simulink model "sampleModel1605_4_sub_sub"  (R2023a)
settings: Solver=VariableStepAuto  StartTime=0.0  StopTime=10.0  RelTol=1e-3
libraries: hdlsllib x2
settings Model: Creator=user1  LastModifiedBy=user1

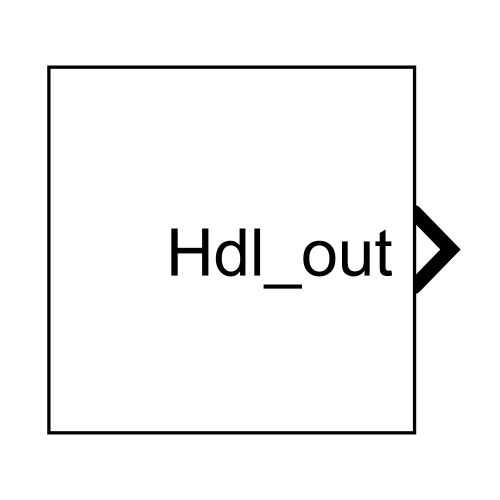
[thumbnail: Simulink's stored preview of the top-level diagram]
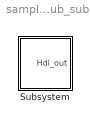
== system sampleModel1605_4_sub_sub ==
  Subsystem : Subsystem

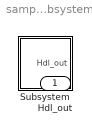
== system sampleModel1605_4_sub_sub/Subsystem ==
  Subsystem : Subsystem
  Hdl_out : Outport  OutDataTypeStr=uint8

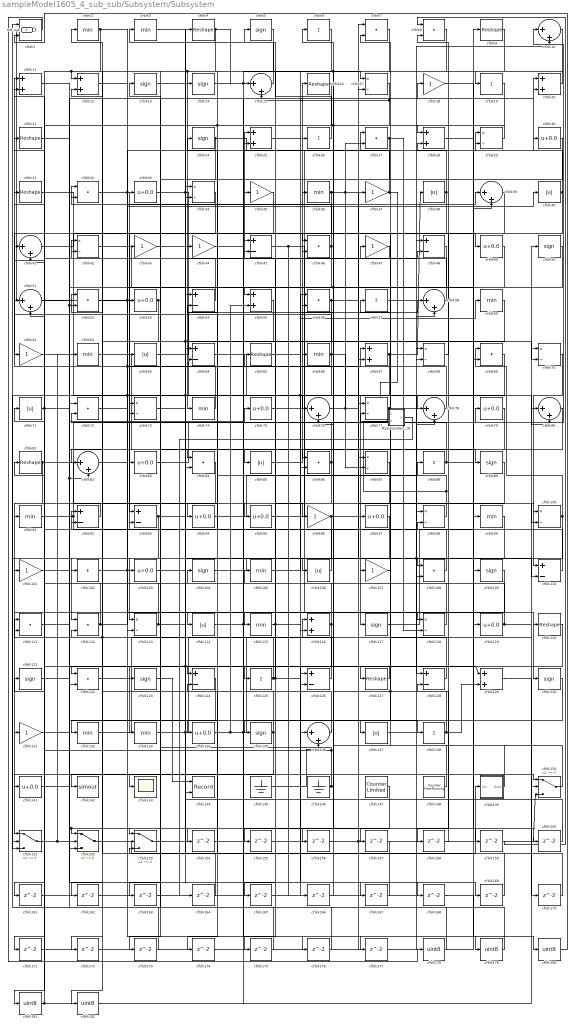
== system sampleModel1605_4_sub_sub/Subsystem/Subsystem ==
  Mysubsystem_16 : Subsystem  TreatAsAtomicUnit=on  RTWFcnName=Mysubsystem_16
      settings: RTWFcnNameOpts=User specified  RTWFileNameOpts=Use function name
  cfblk1 : Logic  AllPortsSameDT=off  OutDataTypeStr=boolean
  cfblk{10,15,39,41,51,58,76,78,80,82,136} (11 alike) : Sum  Inputs=|++  OutDataTypeStr=uint8
  cfblk{17,29,34,42,68,70,73,77,87,98,100,113,118} (13 alike) : Product  Inputs=*/  OutDataTypeStr=uint8  RndMeth=Zero  SaturateOnIntegerOverflow=on
  cfblk{18,35,37,43..44,47,61,96,101,107,131} (11 alike) : Gain  OutDataTypeStr=uint8
  cfblk{6,19,26,57,88,102,125,138} (8 alike) : Sum  Inputs=+  OutDataTypeStr=uint8
  cfblk{30,33,49,53,75,79,83,94..95,97,103,119,134,141} (14 alike) : Bias  Bias=0.0  SaturateOnIntegerOverflow=off
  cfblk{5,13..14,24,50,89,104,109,117,121,123,130,135} (13 alike) : Signum
  cfblk{2..3,36,59,62,66,74,91,99,105,115,132..133} (13 alike) : MinMax  OutDataTypeStr=uint8
  cfblk{38,40,63,71,85,106,114,137} (8 alike) : Abs  OutDataTypeStr=uint8  SaturateOnIntegerOverflow=off
  cfblk{7..8,27,32,46,52,56,69,72,84,86,108,111..112,122} (15 alike) : DotProduct  OutDataTypeStr=uint8
  cfblk{11..12,20,25,28,55,67,116,129} (9 alike) : Sum  OutDataTypeStr=uint8
  cfblk{45,48,54,64,92..93,110,124,126,128} (10 alike) : Sum  Inputs=+-  OutDataTypeStr=uint8
  cfblk{4,9,16,21,31,65,81,120,127} (9 alike) : Reshape
  cfblk142 : ToWorkspace  VariableName=simout  SaveFormat=Timeseries  SampleTime=-1
  cfblk143 : Scope
  cfblk144 : Record  FileSettingsInternal="{\"entries\":[{\"content\":{\"excelSettings\":{\"content\":{},\"type\":\"Streamout.ExcelSettings\"}},\"type\":\"Streamout.FileSettingStorage\",\"uuid\":\"\"}],\"packageUris\":[\"http:\\/\\/schema.mathworks.com\\/mf0\\/streamout_blocks\\/R2020a\"],\"version\":\"1.0\"}"  Layout=[1 1]  SignalsInternal="{\"entries\":[{\"content\":{\"signals\":[{\"content\":{\"blockPath\":[],\"dimensions\":[1],\"domain\":\"\",\"lineColor\":\"#a2142f\",\"plots\":[1],\"port\":1,\"signalID\":29067,\"signalName\":\"cfblk123\"},\"type\":\"RecordBlkView.Signal\",\"uuid\":\"\"},{\"content\":{\"blockPath\":[],\"dimensions\":[1],\"domain\":\"\",\"lineColor\":\"#139fff\",\"plots\":[1],\"port\":2,\"signalID\":29070,\"signalName\":\"cfblk52\"},\"type\":\"RecordBlkView.Signal\",\"uuid\":\"\"}]},\"type\":\"RecordBlkView.InputSignals\",\"uuid\":\"\"}],\"packageUris\":[\"http:\\/\\/schema.mathworks.com\\/mf0\\/streamout_blocks\\/R2020a\"],\"version\":\"1.0\"}"  VisualizationBindings="{\"xyplotplugin\":{\"info\":[{\"series\":[{\"bindingParametersList\":[{\"parameter\":\"X-Axis\",\"signalID\":29067,\"signalName\":\"cfblk123\"},{\"parameter\":\"Y-Axis\",\"signalID\":29070,\"signalName\":\"cfblk52\"}],\"seriesID\":29257}],\"subplotID\":1}]}}"  CompatibilityTag=XY  st=-1
  cfblk145 : Ground
  cfblk146 : Ground
  cfblk147 : hdlsllib/Sources/Counter Limited  uplimit=7  tsamp=-1
  cfblk148 : hdlsllib/Sources/Counter Free-Running  NumBits=16  tsamp=-1
  cfblk149 : Subsystem
      settings: LibrarySourceBlock=|
      | hdlsllib/Ports &
      | Subsystems/Subsystem
  cfblk{150..153} (4 alike) : Switch  OutDataTypeStr=uint8  SaturateOnIntegerOverflow=off  InputSameDT=off
  cfblk{154..177} (24 alike) : Delay  SampleTime=1
  cfblk{178..182} (5 alike) : DataTypeConversion  OutDataTypeStr=uint8  SaturateOnIntegerOverflow=off  RndMeth=Floor
  Hdl_out : Outport  OutDataTypeStr=uint8
  wires:
  Mysubsystem_16/1(Out1) -> cfblk164/1
  cfblk182/1 -> cfblk35/1
  cfblk124/1 -> cfblk182/1
  cfblk181/1 -> cfblk111/2, cfblk80/1
  cfblk180/1 -> cfblk1/2
  cfblk168/1 -> cfblk180/1
  cfblk179/1 -> cfblk1/1
  cfblk154/1 -> cfblk179/1
  cfblk178/1 -> cfblk63/1
  cfblk1/1 -> cfblk178/1
  cfblk177/1 -> cfblk58/2
  cfblk176/1 -> cfblk93/2
  cfblk82/1 -> cfblk176/1
  cfblk175/1 -> cfblk72/1
  cfblk174/1 -> cfblk39/2
  cfblk173/1 -> cfblk11/2
  cfblk79/1 -> cfblk173/1
  cfblk172/1 -> cfblk69/2
  cfblk171/1 -> cfblk17/2
  cfblk170/1 -> cfblk124/2
  cfblk129/1 -> cfblk170/1
  cfblk169/1 -> cfblk54/1
  cfblk101/1 -> cfblk168/1
  cfblk167/1 -> cfblk76/2
  cfblk166/1 -> cfblk56/2
  cfblk165/1 -> cfblk78/2
  cfblk130/1 -> cfblk165/1
  cfblk164/1 -> cfblk112/2
  cfblk163/1 -> cfblk68/2
  cfblk162/1 -> cfblk126/1
  cfblk84/1 -> cfblk162/1
  cfblk161/1 -> cfblk67/2
  cfblk160/1 -> cfblk34/1
  cfblk28/1 -> cfblk160/1
  cfblk159/1 -> cfblk8/1
  cfblk158/1 -> cfblk128/2
  cfblk157/1 -> cfblk153/3
  cfblk25/1 -> cfblk157/1
  cfblk156/1 -> cfblk77/1
  cfblk155/1 -> cfblk7/1
  cfblk87/1 -> cfblk155/1
  cfblk80/1 -> cfblk154/1
  cfblk100/1 -> cfblk151/2, cfblk108/2, cfblk69/1
  cfblk102/1 -> cfblk26/1, cfblk118/1
  cfblk30/1 -> cfblk76/1
  cfblk54/1 -> cfblk32/2
  cfblk148/1 -> cfblk111/1
  cfblk149/1(Out1) -> cfblk105/1
  cfblk136/1 -> cfblk32/1
  cfblk110/1 -> cfblk81/1
  cfblk89/1 -> cfblk107/1
  cfblk98/1 -> Mysubsystem_16/2(In2), cfblk54/2
  cfblk9/1 -> cfblk116/2
  cfblk35/1 -> cfblk181/1
  cfblk4/1 -> cfblk101/1, cfblk15/1
  cfblk46/1 -> cfblk113/2, cfblk12/2
  cfblk72/1 -> cfblk30/1, cfblk64/2
  cfblk76/1 -> cfblk37/1, cfblk27/2, cfblk97/1
  cfblk107/1 -> cfblk77/2
  cfblk69/1 -> cfblk153/2, cfblk151/3
  cfblk3/1 -> cfblk129/1, cfblk169/1, cfblk80/2
  cfblk13/1 -> cfblk70/2, cfblk96/1
  cfblk55/1 -> cfblk84/1
  cfblk97/1 -> cfblk103/1
  cfblk8/1 -> cfblk34/2, cfblk86/1
  cfblk131/1 -> cfblk150/2
  cfblk19/1 -> cfblk141/1
  cfblk92/1 -> cfblk91/1
  cfblk81/1 -> cfblk131/1, cfblk95/1
  cfblk73/1 -> cfblk44/1
  cfblk10/1 -> cfblk125/1
  cfblk12/1 -> cfblk85/1
  cfblk16/1 -> cfblk134/1, cfblk163/1
  cfblk66/1 -> cfblk86/2, cfblk82/1, cfblk51/1, cfblk87/2
  cfblk52/1 -> cfblk144/2, cfblk39/1
  cfblk152/1 -> cfblk149/1(In1)
  cfblk93/1 -> cfblk64/1, cfblk102/1
  cfblk48/1 -> cfblk152/2, cfblk156/1
  cfblk50/1 -> cfblk94/1
  cfblk128/1 -> cfblk7/2
  cfblk68/1 -> cfblk8/2
  cfblk11/1 -> cfblk143/1, cfblk82/2, cfblk52/2
  cfblk113/1 -> cfblk67/1, cfblk92/1
  cfblk120/1 -> cfblk133/1
  cfblk118/1 -> cfblk6/1
  cfblk6/1 -> cfblk132/1
  cfblk117/1 -> cfblk9/1
  cfblk115/1 -> cfblk45/1, cfblk167/1
  cfblk47/1 -> cfblk42/2
  cfblk109/1 -> cfblk151/1
  cfblk126/1 -> cfblk42/1
  cfblk42/1 -> cfblk99/1
  cfblk71/1 -> cfblk31/1, cfblk84/2
  cfblk105/1 -> cfblk59/1
  cfblk32/1 -> cfblk115/1, cfblk27/1
  cfblk145/1 -> cfblk136/2
  cfblk21/1 -> cfblk124/1
  cfblk24/1 -> cfblk29/2, cfblk123/1
  cfblk37/1 -> Mysubsystem_16/1(In1), cfblk25/2
  cfblk94/1 -> cfblk88/1
  cfblk122/1 -> cfblk14/1
  cfblk17/1 -> cfblk46/1, cfblk174/1, cfblk15/2
  cfblk88/1 -> cfblk52/1, cfblk120/1
  cfblk61/1 -> cfblk128/1
  cfblk2/1 -> cfblk12/1, cfblk51/2, cfblk55/1
  cfblk125/1 -> cfblk65/1, cfblk127/1, cfblk92/2, cfblk71/1
  cfblk133/1 -> cfblk70/1, cfblk45/2
  cfblk153/1 -> cfblk87/1, cfblk150/3
  cfblk77/1 -> cfblk72/2, cfblk10/2
  cfblk119/1 -> cfblk50/1, cfblk41/2
  cfblk57/1 -> cfblk48/1
  cfblk103/1 -> cfblk36/1
  cfblk39/1 -> cfblk137/1
  cfblk38/1 -> cfblk135/1, cfblk28/2
  cfblk18/1 -> cfblk119/1
  cfblk74/1 -> cfblk53/1
  cfblk104/1 -> cfblk106/1
  cfblk137/1 -> cfblk68/1
  cfblk59/1 -> cfblk73/1
  cfblk114/1 -> cfblk18/1, cfblk177/1
  cfblk31/1 -> cfblk136/1
  cfblk51/1 -> cfblk98/1
  cfblk63/1 -> cfblk58/1
  cfblk141/1 -> cfblk150/1
  cfblk135/1 -> cfblk2/1, cfblk171/1
  cfblk112/1 -> cfblk40/1, cfblk41/1
  cfblk65/1 -> cfblk56/1
  cfblk41/1 -> cfblk49/1
  cfblk150/1 -> cfblk57/1
  cfblk91/1 -> cfblk79/1, cfblk98/2
  cfblk70/1 -> cfblk110/1
  cfblk116/1 -> cfblk104/1, cfblk161/1
  cfblk43/1 -> cfblk117/1
  cfblk62/1 -> cfblk126/2
  cfblk106/1 -> cfblk24/1
  cfblk111/1 -> cfblk75/1
  cfblk53/1 -> cfblk83/1, Hdl_out/1
  cfblk99/1 -> cfblk112/1
  cfblk20/1 -> cfblk19/1
  cfblk132/1 -> cfblk4/1
  cfblk56/1 -> cfblk142/1, cfblk100/2
  cfblk34/1 -> cfblk61/1
  cfblk121/1 -> cfblk138/1
  cfblk33/1 -> cfblk109/1, cfblk110/2
  cfblk138/1 -> cfblk66/1, cfblk47/1, cfblk129/2
  cfblk146/1 -> cfblk13/1, cfblk121/1, cfblk46/2
  cfblk95/1 -> cfblk29/1
  cfblk14/1 -> cfblk17/1, cfblk159/1
  cfblk96/1 -> cfblk113/1, cfblk100/1
  cfblk44/1 -> cfblk25/1
  cfblk64/1 -> cfblk78/1
  cfblk5/1 -> cfblk114/1
  cfblk49/1 -> cfblk122/2
  cfblk151/1 -> cfblk20/2, cfblk62/1
  cfblk85/1 -> cfblk16/1
  cfblk27/1 -> cfblk153/1, cfblk118/2
  cfblk67/1 -> cfblk38/1, cfblk172/1
  cfblk36/1 -> cfblk93/1, cfblk108/1
  cfblk45/1 -> cfblk130/1, cfblk166/1
  cfblk108/1 -> cfblk33/1
  cfblk40/1 -> cfblk20/1, cfblk158/1
  cfblk127/1 -> cfblk122/1
  cfblk147/1 -> cfblk152/1, cfblk152/3
  cfblk29/1 -> cfblk28/1
  cfblk75/1 -> cfblk89/1
  cfblk86/1 -> cfblk73/2, cfblk175/1
  cfblk26/1 -> cfblk5/1
  cfblk15/1 -> cfblk3/1
  cfblk7/1 -> cfblk74/1, cfblk43/1
  cfblk83/1 -> cfblk10/1
  cfblk58/1 -> cfblk21/1
  cfblk123/1 -> cfblk144/1
  cfblk134/1 -> cfblk116/1, cfblk48/2, cfblk55/2
  cfblk78/1 -> cfblk11/1

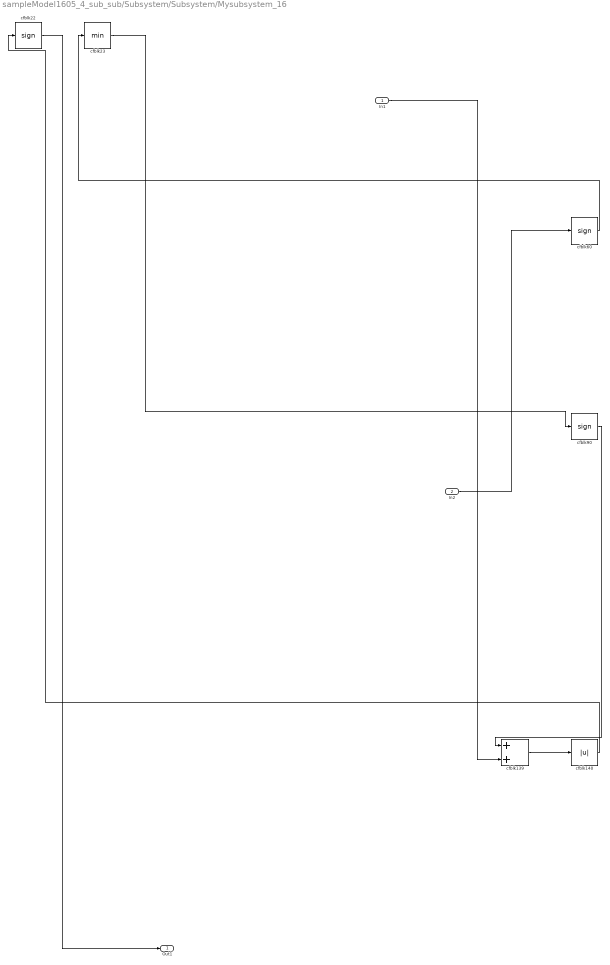
== system sampleModel1605_4_sub_sub/Subsystem/Subsystem/Mysubsystem_16 ==
  In1 : Inport
  In2 : Inport  Port=2
  cfblk139 : Sum
  cfblk140 : Abs  SaturateOnIntegerOverflow=off
  cfblk22 : Signum
  cfblk23 : MinMax
  cfblk60 : Signum
  cfblk90 : Signum
  Out1 : Outport
  wires:
  cfblk60/1 -> cfblk23/1
  cfblk23/1 -> cfblk90/1
  cfblk22/1 -> Out1/1
  cfblk140/1 -> cfblk22/1
  cfblk90/1 -> cfblk139/1
  cfblk139/1 -> cfblk140/1
  In1/1 -> cfblk139/2
  In2/1 -> cfblk60/1

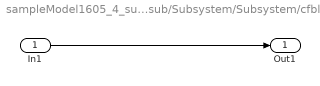
== system sampleModel1605_4_sub_sub/Subsystem/Subsystem/cfblk149 ==
  In1 : Inport
  Out1 : Outport
  wires:
  In1/1 -> Out1/1
